simulink model "machineModel3"  (R2021a)
settings: Solver=VariableStepAuto  StartTime=0.0  StopTime=10.0  RelTol=1e-3
settings Model: Creator=ibirl  LastModifiedBy=ibirl

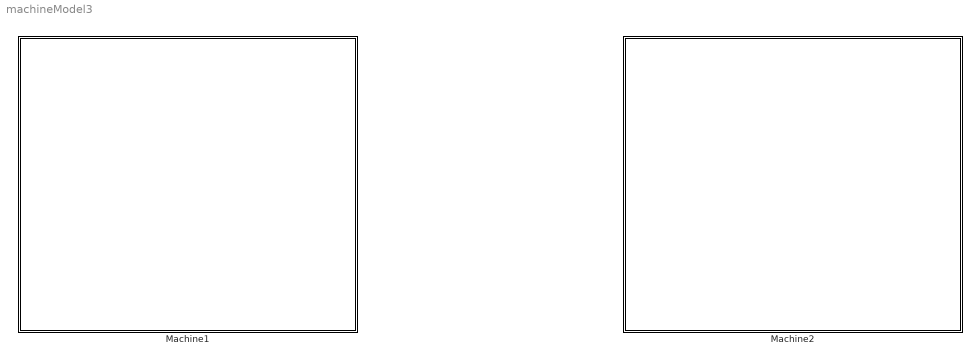
== system machineModel3 ==
  Machine1 : Stateflow chart  TreatAsAtomicUnit=on
  Machine2 : Stateflow chart  TreatAsAtomicUnit=on

== stateflow chart machineModel3/Machine2 ==
  state f
  state e
  state a
  state b
  state c
  state d
  f -> b [order 2] : {0}
  d -> e [order 3] : {-1}
  f -> a [order 1] : {-1}
  f -> e [order 3] : {-1}
  e -> f [order 2] : {0}
  d -> a [order 2] : [1]{-1}
  b -> e [order 3] : {-1}
  e -> e [order 1] : [1]{0}
  c -> e [order 3] : [1]{-1}
  c -> a [order 2] : {-1}
  a -> e [order 3] : {-1}
  b -> a [order 2] : [1]{-1}
  b -> c [order 4] : {0}
  c -> d [order 4] : {0}
  a -> a [order 2] : [1]{-1}
  a -> b [order 1] : {0}
  b -> b [order 1] : {0}
  c -> c [order 1] : {0}
  d -> d [order 1] : {0}

== stateflow chart machineModel3/Machine1 ==
  state I
  state H
  state A
  state B
  state C
  state D
  state E
  state F
  state G
  G -> H [order 3] : {1}
  G -> A [order 2] : [1]{1}
  E -> H [order 3] : {1}
  I -> B [order 2] : {0}
  I -> A [order 1] : {1}
  D -> H [order 3] : {1}
  E -> A [order 4] : {1}
  I -> H [order 3] : {1}
  H -> I [order 2] : {0}
  F -> H [order 4] : {1}
  D -> A [order 4] : {1}
  B -> H [order 3] : {1}
  H -> H [order 1] : [1]{0}
  C -> H [order 4] : [1]{1}
  C -> A [order 3] : {1}
  A -> H [order 3] : {1}
  B -> A [order 2] : [1]{1}
  C -> D [order 1] : {0}
  B -> C [order 4] : {0}
  D -> E [order 1] : {0}
  E -> F [order 1] : {0}
  F -> G [order 1] : {0}
  A -> A [order 2] : [1]{1}
  F -> A [order 3] : {1}
  A -> B [order 1] : {0}
  B -> B [order 1] : {0}
  C -> C [order 2] : {0}
  D -> D [order 2] : {0}
  E -> E [order 2] : {0}
  F -> F [order 2] : {0}
  G -> G [order 1] : {0}
